simulink model "Pacemaker_Assignment_2_Final"  (R2018b)
settings: Solver=FixedStepAuto  StartTime=0.0  StopTime=inf  FixedStep=1e-3  RelTol=1e-3  EnableMultiTasking=on
undefined symbols (not defined in the file): D0, D1, D10, D11, D12, D13, D2, D3, D4, D5, D6, D7, D8, D9, PTA0, PTA1, PTA2, PTB23, PTB9, PTC16, PTC17, PTC2, PTC3, PTC4, PTD0, PTD1, PTD2, PTD3
libraries: frdmk64flib x20, dspstat3 x1
(part 2 of 2)

== stateflow chart Pacemaker_Assignment_2_Final/Pacing ==
  state VOO
    note: VOO just paces the ventricle at a rate predetermined by the LRL. Charging and discharging are seperate states simply for the sake of making the model visually similar
        | to the pacemaker shield explained doc's description of pulsing
    state Start
      entry:
      VOO_Charge_Time = 60000/Lower_Rate_Limit - Ventricular_Pulse_Width;
    state Pacing_Ventricle
      entry:
      PACE_CHARGE_CTRL = false;
      PACE_GND_CTRL = true;
      ATR_PACE_CTRL = false;
      ATR_GND_CTRL = false;
      Z_ATR_CTRL = false;
      Z_VENT_CTRL = false;
      VENT_GND_CTRL = false;
      VENT_PACE_CTRL = true;
    state Discharge_Ventricle
      entry:
      PACE_GND_CTRL = true;
      VENT_PACE_CTRL = false;
      Z_ATR_CTRL = false;
      Z_VENT_CTRL = false;
      ATR_PACE_CTRL = false;
      ATR_GND_CTRL = false;
      VENT_GND_CTRL = true;
    state Charging_Ventricle
      entry:
      ATR_PACE_CTRL = false;
      VENT_PACE_CTRL = false;
      PACING_REF_PWM = Ventricular_PWM;
      PACE_CHARGE_CTRL = true;
    (default) -> VOO.Start
    VOO.Start -> VOO.Charging_Ventricle
    VOO.Charging_Ventricle -> VOO.Pacing_Ventricle : [after(VOO_Charge_Time, msec)]
    VOO.Pacing_Ventricle -> VOO.Discharge_Ventricle : [after(Ventricular_Pulse_Width, msec)]
    VOO.Discharge_Ventricle -> VOO.Charging_Ventricle
  state AAI
    note: AAI still paces the atrium like AOO did, but must also inhibit the pacemaker if it senses a natural pace after the atrial refractory period has been reached since the last pulse (paced/natural)
    state Start
      entry:
      AAI_Charge_Time = 60000/Lower_Rate_Limit - Atrial_Pulse_Width;
      FRONTEND_CTRL = true;
    state Pacing_Atrial
      entry:
      PACE_CHARGE_CTRL = false;
      PACE_GND_CTRL = true;
      ATR_PACE_CTRL = true;
      ATR_GND_CTRL = false;
      Z_ATR_CTRL = false;
      Z_VENT_CTRL = false;
      VENT_GND_CTRL = false;
      VENT_PACE_CTRL = false;
    state Discharge_Atrial
      entry:
      PACE_GND_CTRL = true;
      VENT_PACE_CTRL = false;
      Z_ATR_CTRL = false;
      Z_VENT_CTRL = false;
      ATR_PACE_CTRL = false;
      ATR_GND_CTRL = true;
      VENT_GND_CTRL = false;
    state Charging_Atrial
      entry:
      ATR_PACE_CTRL = false;
      VENT_PACE_CTRL = false;
      PACING_REF_PWM = Atrial_PWM;
      PACE_CHARGE_CTRL = true;
    (default) -> AAI.Start
    AAI.Charging_Atrial -> AAI.Discharge_Atrial [order 2] : [Atrial_Pulse && after(ARP, msec)]
    AAI.Start -> AAI.Charging_Atrial
    AAI.Charging_Atrial -> AAI.Pacing_Atrial [order 1] : [after(AAI_Charge_Time, msec)]
    AAI.Pacing_Atrial -> AAI.Discharge_Atrial : [after(Atrial_Pulse_Width, msec)]
    AAI.Discharge_Atrial -> AAI.Charging_Atrial
  state VVI
    note: VVI still paces the atrium like VOO did, but must also inhibit the pacemaker if it senses a natural pace after the ventricular refractory period has been reached since the last pulse (paced/natural)
    state Start
      entry:
      VVI_Charge_Time = 60000/Lower_Rate_Limit - Ventricular_Pulse_Width;
      FRONTEND_CTRL = true;
    state Pacing_Ventricle
      entry:
      PACE_CHARGE_CTRL = false;
      PACE_GND_CTRL = true;
      ATR_PACE_CTRL = false;
      ATR_GND_CTRL = false;
      Z_ATR_CTRL = false;
      Z_VENT_CTRL = false;
      VENT_GND_CTRL = false;
      VENT_PACE_CTRL = true;
    state Discharge_Ventricle
      entry:
      PACE_GND_CTRL = true;
      VENT_PACE_CTRL = false;
      Z_ATR_CTRL = false;
      Z_VENT_CTRL = false;
      ATR_PACE_CTRL = false;
      ATR_GND_CTRL = false;
      VENT_GND_CTRL = true;
    state Charging_Ventricle
      entry:
      ATR_PACE_CTRL = false;
      VENT_PACE_CTRL = false;
      PACING_REF_PWM = Ventricular_PWM;
      PACE_CHARGE_CTRL = true;
    (default) -> VVI.Start
    VVI.Charging_Ventricle -> VVI.Discharge_Ventricle [order 2] : [Ventricular_Pulse && after(VRP, msec)]
    VVI.Start -> VVI.Charging_Ventricle
    VVI.Pacing_Ventricle -> VVI.Discharge_Ventricle : [after(Ventricular_Pulse_Width, msec)]
    VVI.Charging_Ventricle -> VVI.Pacing_Ventricle [order 1] : [after(VVI_Charge_Time, msec)]
    VVI.Discharge_Ventricle -> VVI.Charging_Ventricle
  note: Mode
      | Enum
      |
      | AOO
      | 1
      |
      | VOO
      | 2
      |
      | AAI
      | 3
      |
      | VVI
      | 4
      |
      | DOO
      | 5
      |
      | AOOR
      | 6
      |
      | VOOR
      | 7
      |
      | AAIR
      | 8
      |
      | VVIR
      | 9
      |
      | DOOR
      | 10
  state AOO
    note: AOO just paces the atrium at a rate predetermined by the LRL. Charging and discharging are seperate states simply for the sake of making the model visually similar
        | to the pacemaker shield explained doc's description of pulsing
    state Start
      entry:
      AOO_Charge_Time = 60000/Lower_Rate_Limit - Atrial_Pulse_Width;
    state Pacing_Atrium
      entry:
      PACE_CHARGE_CTRL = false;
      PACE_GND_CTRL = true;
      ATR_PACE_CTRL = true;
      ATR_GND_CTRL = false;
      Z_ATR_CTRL = false;
      Z_VENT_CTRL = false;
      VENT_GND_CTRL = false;
      VENT_PACE_CTRL = false;
    state Discharge_Atrium
      entry:
      PACE_GND_CTRL = true;
      VENT_PACE_CTRL = false;
      Z_ATR_CTRL = false;
      Z_VENT_CTRL = false;
      ATR_PACE_CTRL = false;
      ATR_GND_CTRL = true;
      VENT_GND_CTRL = false;
    state Charging_Atrium
      entry:
      ATR_PACE_CTRL = false;
      VENT_PACE_CTRL = false;
      PACING_REF_PWM = Atrial_PWM;
      PACE_CHARGE_CTRL = true;
    (default) -> AOO.Start
    AOO.Start -> Charging_Atrium
    Charging_Atrium -> Pacing_Atrium : [after(AOO_Charge_Time, msec)]
    Pacing_Atrium -> Discharge_Atrium : [after(Atrial_Pulse_Width, msec)]
    Discharge_Atrium -> Charging_Atrium
  state DOO
    state Start
      entry:
      DOO_Charge_Time = 60000/Lower_Rate_Limit - Fixed_AV_Delay - Ventricular_Pulse_Width;
      DOO_AV_Delay = Fixed_AV_Delay - Atrial_Pulse_Width;
      %Fixed AV Delay is from start of atrial pulse to start of ventricular pulse (must include atrial pulse width time)
    note: DOO pulses the atrium and ventricle using the LRL and Fixed AV delay for timing. The mode
        | simply transitions from pacing the ventricle to pacing the atrium and then repeats. For this mode
        | pulse amplitude sent can vary for the chambers so it must be changed based on the chamber.
    state Pacing_Ventricle
      entry:
      PACE_CHARGE_CTRL = false;
      PACE_GND_CTRL = true;
      ATR_PACE_CTRL = false;
      ATR_GND_CTRL = false;
      Z_ATR_CTRL = false;
      Z_VENT_CTRL = false;
      VENT_GND_CTRL = false;
      VENT_PACE_CTRL = true;
    state Discharge_Ventricle
      entry:
      PACE_GND_CTRL = true;
      VENT_PACE_CTRL = false;
      Z_ATR_CTRL = false;
      Z_VENT_CTRL = false;
      ATR_PACE_CTRL = false;
      ATR_GND_CTRL = false;
      VENT_GND_CTRL = true;
    state Charging_Ventricle
      entry:
      ATR_PACE_CTRL = false;
      VENT_PACE_CTRL = false;
      PACING_REF_PWM = Ventricular_PWM;
      PACE_CHARGE_CTRL = true;
    state Discharge_Atrial
      entry:
      PACE_GND_CTRL = true;
      VENT_PACE_CTRL = false;
      Z_ATR_CTRL = false;
      Z_VENT_CTRL = false;
      ATR_PACE_CTRL = false;
      ATR_GND_CTRL = true;
      VENT_GND_CTRL = false;
    state Pacing_Atrial
      entry:
      PACE_CHARGE_CTRL = false;
      PACE_GND_CTRL = true;
      ATR_PACE_CTRL = true;
      ATR_GND_CTRL = false;
      Z_ATR_CTRL = false;
      Z_VENT_CTRL = false;
      VENT_GND_CTRL = false;
      VENT_PACE_CTRL = false;
    state Charging_Atrial
      entry:
      ATR_PACE_CTRL = false;
      VENT_PACE_CTRL = false;
      PACING_REF_PWM = Atrial_PWM;
      PACE_CHARGE_CTRL = true;
    (default) -> DOO.Start
    DOO.Start -> DOO.Charging_Ventricle
    DOO.Charging_Ventricle -> DOO.Pacing_Ventricle : [after(DOO_AV_Delay, msec)]
    DOO.Pacing_Ventricle -> DOO.Discharge_Ventricle : [after(Ventricular_Pulse_Width, msec)]
    DOO.Discharge_Atrial -> DOO.Charging_Ventricle
    DOO.Discharge_Ventricle -> DOO.Charging_Atrial
    DOO.Pacing_Atrial -> DOO.Discharge_Atrial : [after(Atrial_Pulse_Width, msec)]
    DOO.Charging_Atrial -> DOO.Pacing_Atrial : [after(DOO_Charge_Time, msec)]
  state Mode %Go to mode (allows mode transition by serial)
    entry: %Set PWM values, range in rates
    Atrial_PWM = 100*Atrial_Amplitude/5;
    Ventricular_PWM = 100*Ventricular_Amplitude/5;
    Rate_Range = Max_Sensor_Rate - Lower_Rate_Limit;
    K = 3; %Arbitrary Constant (Range of Activity at RF = 1)
    ATR_PACE_CTRL = false;
    VENT_PACE_CTRL = false;
  state DOOR
    note: Rate Increase = (MSR-LRL)/Reaction Time
        | Rate Decrease = (MSR-LRL)/Recovery Time
        | Rate Range = MSR - LRL
        | Target Rate = LRL + Response Factor * (MSR - LRL)/K*(Activity - Activity Threshold)
        | Target Constant = Response Factor * Rate Range / K
        | Target Rate = LRL + Target Constant * (Activity - Activity Threshold)
    state Pacing_Ventricle
      entry:
      PACE_CHARGE_CTRL = false;
      PACE_GND_CTRL = true;
      ATR_PACE_CTRL = false;
      ATR_GND_CTRL = false;
      Z_ATR_CTRL = false;
      Z_VENT_CTRL = false;
      VENT_GND_CTRL = false;
      VENT_PACE_CTRL = true;
    state Discharge_Ventricle
      entry:
      PACE_GND_CTRL = true;
      VENT_PACE_CTRL = false;
      Z_ATR_CTRL = false;
      Z_VENT_CTRL = false;
      ATR_PACE_CTRL = false;
      ATR_GND_CTRL = false;
      VENT_GND_CTRL = true;
    state Charging_Atrial
      entry:
      ATR_PACE_CTRL = false;
      VENT_PACE_CTRL = false;
      PACING_REF_PWM = Atrial_PWM;
      PACE_CHARGE_CTRL = true;
    state Start
      entry:
      DOOR_AV_Delay = Fixed_AV_Delay - Atrial_Pulse_Width;
      %Fixed AV Delay is from start of atrial pulse to start of ventricular pulse (must include atrial pulse width time)
      DOOR_Rate = Lower_Rate_Limit;
      DOOR_Target = Lower_Rate_Limit; %Need to initialize
      Rate_Increase = (Rate_Range) / Reaction_Time;
      Rate_Decrease = (Rate_Range) / Recovery_Time;
      Target_Constant = Response_Factor * Rate_Range/K;
    state Charging_Ventricle
      entry:
      ATR_PACE_CTRL = false;
      VENT_PACE_CTRL = false;
      PACING_REF_PWM = Ventricular_PWM;
      PACE_CHARGE_CTRL = true;
      DOOR_Interval = 60000/DOOR_Rate - DOOR_AV_Delay - Ventricular_Pulse_Width;
      %Interval is calculated every loop incase rate changes
    state Pacing_Atrial
      entry:
      PACE_CHARGE_CTRL = false;
      PACE_GND_CTRL = true;
      ATR_PACE_CTRL = true;
      ATR_GND_CTRL = false;
      Z_ATR_CTRL = false;
      Z_VENT_CTRL = false;
      VENT_GND_CTRL = false;
      VENT_PACE_CTRL = false;
    state Discharge_Atrial
      entry:
      PACE_GND_CTRL = true;
      VENT_PACE_CTRL = false;
      Z_ATR_CTRL = false;
      Z_VENT_CTRL = false;
      ATR_PACE_CTRL = false;
      ATR_GND_CTRL = true;
      VENT_GND_CTRL = false;
    state Active
      entry:
      DOOR_Target = Lower_Rate_Limit + Target_Constant*(Activity - Activity_Threshold);
      DOOR_Target = min(Max_Sensor_Rate, DOOR_Target);
      %Ensure target rate is below max sensor rate
      Smooth_Rate_Increase = DOOR_Rate * Rate_Smoothing_Up/100;
    state Increase_Rate
      entry:
      DOOR_Increase = min(Smooth_Rate_Increase, Rate_Increase);
      %Applies Rate Smoothing
      DOOR_Increase = DOOR_Increase * 60/DOOR_Rate;
      DOOR_Rate = DOOR_Rate + DOOR_Increase;
    state Rate_Adaptive
      %Determines branch based on activity relative to threshold
      %Must be 0.1g above or below threshold to adjust rate
    state Limit_Rate
      %Ensure rate is between target and LRL
      entry:
      DOOR_Rate = min(DOOR_Target, DOOR_Rate);
      DOOR_Rate = max(Lower_Rate_Limit, DOOR_Rate);
    state Inactive
      entry:
      Smooth_Rate_Decrease = AAIR_Rate * Rate_Smoothing_Down/100;
    state Decrease_Rate
      entry:
      DOOR_Decrease = min(Smooth_Rate_Decrease, Rate_Decrease);
      %Applies Rate Smoothing
      DOOR_Decrease = DOOR_Decrease * 60/DOOR_Rate;
      DOOR_Rate = DOOR_Rate - DOOR_Decrease;
    (default) -> DOOR.Start
    DOOR.Charging_Ventricle -> DOOR.Pacing_Ventricle : [after(DOOR_AV_Delay, msec)]
    DOOR.Discharge_Ventricle -> DOOR.Charging_Atrial
    DOOR.Pacing_Ventricle -> DOOR.Discharge_Ventricle : [after(Ventricular_Pulse_Width, msec)]
    DOOR.Charging_Atrial -> DOOR.Pacing_Atrial : [after(DOOR_Interval, msec)]
    DOOR.Start -> DOOR.Charging_Ventricle
    DOOR.Limit_Rate -> DOOR.Charging_Ventricle
    DOOR.Pacing_Atrial -> DOOR.Discharge_Atrial : [after(Atrial_Pulse_Width, msec)]
    DOOR.Discharge_Atrial -> DOOR.Rate_Adaptive
    DOOR.Active -> DOOR.Increase_Rate
    DOOR.Rate_Adaptive -> DOOR.Active [order 1] : [Activity > (Activity_Threshold + 0.1)]
    DOOR.Increase_Rate -> DOOR.Limit_Rate
    DOOR.Rate_Adaptive -> DOOR.Limit_Rate [order 3] : [(Activity <= (Activity_Threshold + 0.1)) && (Activity >= (Activity_Threshold - 0.1))]
    DOOR.Rate_Adaptive -> DOOR.Inactive [order 2] : [Activity < (Activity_Threshold - 0.1)]
    DOOR.Decrease_Rate -> DOOR.Limit_Rate
    DOOR.Inactive -> DOOR.Decrease_Rate
  state AOOR
    note: Rate Increase = (MSR-LRL)/Reaction Time
        | Rate Decrease = (MSR-LRL)/Recovery Time
        | Rate Range = MSR - LRL
        | Target Rate = LRL + Response Factor * (MSR - LRL)/K*(Activity - Activity Threshold)
        | Target Constant = Response Factor * Rate Range / K
        | Target Rate = LRL + Target Constant * (Activity - Activity Threshold)
    state Start
      entry:
      AOOR_Rate = Lower_Rate_Limit;
      AOOR_Target = Lower_Rate_Limit; %Need to initialize
      Rate_Increase = (Rate_Range) / Reaction_Time;
      Rate_Decrease = (Rate_Range) / Recovery_Time;
      Target_Constant = Response_Factor * Rate_Range/K;
    state Pacing_Atrial
      entry:
      PACE_CHARGE_CTRL = false;
      PACE_GND_CTRL = true;
      ATR_PACE_CTRL = true;
      ATR_GND_CTRL = false;
      Z_ATR_CTRL = false;
      Z_VENT_CTRL = false;
      VENT_GND_CTRL = false;
      VENT_PACE_CTRL = false;
    state Discharge_Atrial
      entry:
      PACE_GND_CTRL = true;
      VENT_PACE_CTRL = false;
      Z_ATR_CTRL = false;
      Z_VENT_CTRL = false;
      ATR_PACE_CTRL = false;
      ATR_GND_CTRL = true;
      VENT_GND_CTRL = false;
    state Charging_Atrial
      entry:
      ATR_PACE_CTRL = false;
      VENT_PACE_CTRL = false;
      PACING_REF_PWM = Atrial_PWM;
      PACE_CHARGE_CTRL = true;
      AOOR_Interval = 60000/AOOR_Rate - Atrial_Pulse_Width;
      %Interval is calculated every loop incase rate changes
    state Active
      entry:
      AOOR_Target = Lower_Rate_Limit + Target_Constant*(Activity - Activity_Threshold);
      AOOR_Target = min(Max_Sensor_Rate, AOOR_Target);
      %Ensure target rate is below max sensor rate
      Smooth_Rate_Increase = AOOR_Rate * Rate_Smoothing_Up/100;
    state Increase_Rate
      entry:
      AOOR_Increase = min(Smooth_Rate_Increase, Rate_Increase);
      %Applies Rate Smoothing
      AOOR_Increase = AOOR_Increase * 60/AOOR_Rate;
      AOOR_Rate = AOOR_Rate + AOOR_Increase;
    state Rate_Adaptive
      %Determines branch based on activity relative to threshold
      %Must be 0.1g above or below threshold to adjust rate
    state Limit_Rate
      %Ensure rate is between target and LRL
      entry:
      AOOR_Rate = min(AOOR_Target, AOOR_Rate);
      AOOR_Rate = max(Lower_Rate_Limit, AOOR_Rate);
    state Inactive
      entry:
      Smooth_Rate_Decrease = AAIR_Rate * Rate_Smoothing_Down/100;
    state Decrease_Rate
      entry:
      AOOR_Decrease = min(Smooth_Rate_Decrease, Rate_Decrease);
      %Applies Rate Smoothing
      AOOR_Decrease = AOOR_Decrease * 60/AOOR_Rate;
      AOOR_Rate = AOOR_Rate - AOOR_Decrease;
    (default) -> AOOR.Start
    AOOR.Start -> AOOR.Charging_Atrial
    AOOR.Charging_Atrial -> AOOR.Pacing_Atrial : [after(AOOR_Interval, msec)]
    AOOR.Pacing_Atrial -> AOOR.Discharge_Atrial : [after(Atrial_Pulse_Width, msec)]
    AOOR.Limit_Rate -> AOOR.Charging_Atrial
    AOOR.Discharge_Atrial -> AOOR.Rate_Adaptive
    AOOR.Active -> AOOR.Increase_Rate
    AOOR.Rate_Adaptive -> AOOR.Active [order 1] : [Activity > (Activity_Threshold + 0.1)]
    AOOR.Increase_Rate -> AOOR.Limit_Rate
    AOOR.Rate_Adaptive -> AOOR.Limit_Rate [order 3] : [(Activity <= (Activity_Threshold + 0.1)) && (Activity >= (Activity_Threshold - 0.1))]
    AOOR.Rate_Adaptive -> AOOR.Inactive [order 2] : [Activity < (Activity_Threshold - 0.1)]
    AOOR.Decrease_Rate -> AOOR.Limit_Rate
    AOOR.Inactive -> AOOR.Decrease_Rate
  note: This is where common variables between modes are set, and the pacemaker mode is determined. This design allows hiding of the mode implementations and allows a more modular device. This setup also ensures that a mode is left once the mode changes (==mode to enter, ~= mode to exit).
  state VVIR
    state Start
      entry:
      VVIR_Rate = Lower_Rate_Limit;
      VVIR_Target = Lower_Rate_Limit; %Need to initialize
      Rate_Increase = (Rate_Range) / Reaction_Time;
      Rate_Decrease = (Rate_Range) / Recovery_Time;
      Target_Constant = Response_Factor * Rate_Range/K;
      FRONTEND_CTRL = true;
    note: Rate Increase = (MSR-LRL)/Reaction Time
        | Rate Decrease = (MSR-LRL)/Recovery Time
        | Rate Range = MSR - LRL
        | Target Rate = LRL + Response Factor * (MSR - LRL)/K*(Activity - Activity Threshold)
        | Target Constant = Response Factor * Rate Range / K
        | Target Rate = LRL + Target Constant * (Activity - Activity Threshold)
    state Charging_Ventricle
      entry:
      ATR_PACE_CTRL = false;
      VENT_PACE_CTRL = false;
      PACING_REF_PWM = Ventricular_PWM;
      PACE_CHARGE_CTRL = true;
      VVIR_Interval = 60000/VVIR_Rate - Ventricular_Pulse_Width;
      %Interval is calculated every loop incase rate changes
      sensed = false;
    state Pacing_Ventricle
      entry:
      PACE_CHARGE_CTRL = false;
      PACE_GND_CTRL = true;
      ATR_PACE_CTRL = false;
      ATR_GND_CTRL = false;
      Z_ATR_CTRL = false;
      Z_VENT_CTRL = false;
      VENT_GND_CTRL = false;
      VENT_PACE_CTRL = true;
    state Discharge_Ventricle
      entry:
      PACE_GND_CTRL = true;
      VENT_PACE_CTRL = false;
      Z_ATR_CTRL = false;
      Z_VENT_CTRL = false;
      ATR_PACE_CTRL = false;
      ATR_GND_CTRL = false;
      VENT_GND_CTRL = true;
    state Increase_Rate_Sensed
      entry:
      VVIR_Increase = min(Smooth_Rate_Increase, Rate_Increase);
      %Applies Rate Smoothing
      VVIR_Increase = VVIR_Increase * VRP/1000;
      VVIR_Rate = VVIR_Rate + VVIR_Increase;
    state Active
      entry:
      VVIR_Target = Lower_Rate_Limit + Target_Constant*(Activity - Activity_Threshold);
      VVIR_Target = min(Max_Sensor_Rate, VVIR_Target);
      %Ensure target rate is below max sensor rate
      Smooth_Rate_Increase = VVIR_Rate * Rate_Smoothing_Up/100;
    state Increase_Rate_Paced
      entry:
      VVIR_Increase = min(Smooth_Rate_Increase, Rate_Increase);
      %Applies Rate Smoothing
      VVIR_Increase = VVIR_Increase * 60/VVIR_Rate;
      VVIR_Rate = VVIR_Rate + VVIR_Increase;
    state Rate_Adaptive
      %Determines branch based on activity relative to threshold
      %Must be 0.1g above or below threshold to adjust rate
    state Limit_Rate
      %Ensure rate is between target and LRL
      entry:
      VVIR_Rate = min(VVIR_Target, VVIR_Rate);
      VVIR_Rate = max(Lower_Rate_Limit, VVIR_Rate);
    state Decrease_Rate_Sensed
      entry:
      VVIR_Decrease = min(Smooth_Rate_Decrease, Rate_Decrease);
      %Applies Rate Smoothing
      VVIR_Decrease = VVIR_Decrease * VRP/1000;
      VVIR_Rate = VVIR_Rate - VVIR_Decrease;
    state Inactive
      entry:
      Smooth_Rate_Decrease = VVIR_Rate * Rate_Smoothing_Down/100;
    state Decrease_Rate_Paced
      entry:
      VVIR_Decrease = min(Smooth_Rate_Decrease, Rate_Decrease);
      %Applies Rate Smoothing
      VVIR_Decrease = VVIR_Decrease * 60/VVIR_Rate;
      VVIR_Rate = VVIR_Rate - VVIR_Decrease;
    (default) -> VVIR.Start
    VVIR.Start -> VVIR.Charging_Ventricle
    VVIR.Charging_Ventricle -> VVIR.Discharge_Ventricle [order 1] : [Ventricular_Pulse && after(VRP, msec)]{sensed = true;}
    VVIR.Charging_Ventricle -> VVIR.Pacing_Ventricle [order 2] : [after(VVIR_Interval, msec)]
    VVIR.Pacing_Ventricle -> VVIR.Discharge_Ventricle : [after(Ventricular_Pulse_Width, msec)]
    VVIR.Limit_Rate -> VVIR.Charging_Ventricle
    VVIR.Discharge_Ventricle -> VVIR.Rate_Adaptive
    VVIR.Active -> VVIR.Increase_Rate_Sensed [order 1] : [sensed]
    VVIR.Increase_Rate_Sensed -> VVIR.Limit_Rate
    VVIR.Rate_Adaptive -> VVIR.Active [order 1] : [Activity > (Activity_Threshold + 0.1)]
    VVIR.Active -> VVIR.Increase_Rate_Paced [order 2] : [~sensed]
    VVIR.Increase_Rate_Paced -> VVIR.Limit_Rate
    VVIR.Rate_Adaptive -> VVIR.Limit_Rate [order 3] : [(Activity <= (Activity_Threshold + 0.1)) && (Activity >= (Activity_Threshold - 0.1))]
    VVIR.Decrease_Rate_Sensed -> VVIR.Limit_Rate
    VVIR.Rate_Adaptive -> VVIR.Inactive [order 2] : [Activity < (Activity_Threshold - 0.1)]
    VVIR.Decrease_Rate_Paced -> VVIR.Limit_Rate
    VVIR.Inactive -> VVIR.Decrease_Rate_Sensed [order 2] : [sensed]
    VVIR.Inactive -> VVIR.Decrease_Rate_Paced [order 1] : [~sensed]
  state AAIR
    note: Rate Increase = (MSR-LRL)/Reaction Time
        | Rate Decrease = (MSR-LRL)/Recovery Time
        | Rate Range = MSR - LRL
        | Target Rate = LRL + Response Factor * (MSR - LRL)/K*(Activity - Activity Threshold)
        | Target Constant = Response Factor * Rate Range / K
        | Target Rate = LRL + Target Constant * (Activity - Activity Threshold)
    state Start
      entry:
      AAIR_Rate = Lower_Rate_Limit;
      AAIR_Target = Lower_Rate_Limit; %Need to initialize
      Rate_Increase = (Rate_Range) / Reaction_Time;
      Rate_Decrease = (Rate_Range) / Recovery_Time;
      Target_Constant = Response_Factor * Rate_Range/K;
      FRONTEND_CTRL = true;
    state Charging_Atrial
      entry:
      ATR_PACE_CTRL = false;
      VENT_PACE_CTRL = false;
      PACING_REF_PWM = Atrial_PWM;
      PACE_CHARGE_CTRL = true;
      AAIR_Interval = 60000/AAIR_Rate - Atrial_Pulse_Width;
      %Interval is calculated every loop incase rate changes
      sensed = false;
    state Pacing_Atrial
      entry:
      PACE_CHARGE_CTRL = false;
      PACE_GND_CTRL = true;
      ATR_PACE_CTRL = true;
      ATR_GND_CTRL = false;
      Z_ATR_CTRL = false;
      Z_VENT_CTRL = false;
      VENT_GND_CTRL = false;
      VENT_PACE_CTRL = false;
    state Discharge_Atrial
      entry:
      PACE_GND_CTRL = true;
      VENT_PACE_CTRL = false;
      Z_ATR_CTRL = false;
      Z_VENT_CTRL = false;
      ATR_PACE_CTRL = false;
      ATR_GND_CTRL = true;
      VENT_GND_CTRL = false;
    state Increase_Rate_Sensed
      entry:
      AAIR_Increase = min(Smooth_Rate_Increase, Rate_Increase);
      %Applies Rate Smoothing
      AAIR_Increase = AAIR_Increase * ARP/1000;
      AAIR_Rate = AAIR_Rate + AAIR_Increase;
    state Active
      entry:
      AAIR_Target = Lower_Rate_Limit + Target_Constant*(Activity - Activity_Threshold);
      AAIR_Target = min(Max_Sensor_Rate, AAIR_Target);
      %Ensure target rate is below max sensor rate
      Smooth_Rate_Increase = AAIR_Rate * Rate_Smoothing_Up/100;
    state Increase_Rate_Paced
      entry:
      AAIR_Increase = min(Smooth_Rate_Increase, Rate_Increase);
      %Applies Rate Smoothing
      AAIR_Increase = AAIR_Increase * 60/AAIR_Rate;
      AAIR_Rate = AAIR_Rate + AAIR_Increase;
    state Rate_Adaptive
      %Determines branch based on activity relative to threshold
      %Must be 0.1g above or below threshold to adjust rate
    state Limit_Rate
      %Ensure rate is between target and LRL
      entry:
      AAIR_Rate = min(AAIR_Target, AAIR_Rate);
      AAIR_Rate = max(Lower_Rate_Limit, AAIR_Rate);
    state Decrease_Rate_Sensed
      entry:
      AAIR_Decrease = min(Smooth_Rate_Decrease, Rate_Decrease);
      %Applies Rate Smoothing
      AAIR_Decrease = AAIR_Decrease * ARP/1000;
      AAIR_Rate = AAIR_Rate - AAIR_Decrease;
    state Inactive
      entry:
      Smooth_Rate_Decrease = AAIR_Rate * Rate_Smoothing_Down/100;
    state Decrease_Rate_Paced
      entry:
      AAIR_Decrease = min(Smooth_Rate_Decrease, Rate_Decrease);
      %Applies Rate Smoothing
      AAIR_Decrease = AAIR_Decrease * 60/AAIR_Rate;
      AAIR_Rate = AAIR_Rate - AAIR_Decrease;
    (default) -> AAIR.Start
    AAIR.Charging_Atrial -> AAIR.Discharge_Atrial [order 1] : [Atrial_Pulse && after(ARP, msec)]{sensed = true;}
    AAIR.Start -> AAIR.Charging_Atrial
    AAIR.Charging_Atrial -> AAIR.Pacing_Atrial [order 2] : [after(AAIR_Interval, msec)]
    AAIR.Pacing_Atrial -> AAIR.Discharge_Atrial : [after(Atrial_Pulse_Width, msec)]
    AAIR.Limit_Rate -> AAIR.Charging_Atrial
    AAIR.Discharge_Atrial -> AAIR.Rate_Adaptive
    AAIR.Active -> AAIR.Increase_Rate_Sensed [order 1] : [sensed]
    AAIR.Increase_Rate_Sensed -> AAIR.Limit_Rate
    AAIR.Rate_Adaptive -> AAIR.Active [order 1] : [Activity > (Activity_Threshold + 0.1)]
    AAIR.Active -> AAIR.Increase_Rate_Paced [order 2] : [~sensed]
    AAIR.Increase_Rate_Paced -> AAIR.Limit_Rate
    AAIR.Rate_Adaptive -> AAIR.Limit_Rate [order 3] : [(Activity <= (Activity_Threshold + 0.1)) && (Activity >= (Activity_Threshold - 0.1))]
    AAIR.Decrease_Rate_Sensed -> AAIR.Limit_Rate
    AAIR.Rate_Adaptive -> AAIR.Inactive [order 2] : [Activity < (Activity_Threshold - 0.1)]
    AAIR.Decrease_Rate_Paced -> AAIR.Limit_Rate
    AAIR.Inactive -> AAIR.Decrease_Rate_Sensed [order 2] : [sensed]
    AAIR.Inactive -> AAIR.Decrease_Rate_Paced [order 1] : [~sensed]
  state VOOR
    state Start
      entry:
      VOOR_Rate = Lower_Rate_Limit;
      VOOR_Target = Lower_Rate_Limit; %Need to initialize
      Rate_Increase = (Rate_Range) / Reaction_Time;
      Rate_Decrease = (Rate_Range) / Recovery_Time;
      Target_Constant = Response_Factor * Rate_Range/K;
    note: Rate Increase = (MSR-LRL)/Reaction Time
        | Rate Decrease = (MSR-LRL)/Recovery Time
        | Rate Range = MSR - LRL
        | Target Rate = LRL + Response Factor * (MSR - LRL)/K*(Activity - Activity Threshold)
        | Target Constant = Response Factor * Rate Range / K
        | Target Rate = LRL + Target Constant * (Activity - Activity Threshold)
    state Pacing_Ventricle
      entry:
      PACE_CHARGE_CTRL = false;
      PACE_GND_CTRL = true;
      ATR_PACE_CTRL = false;
      ATR_GND_CTRL = false;
      Z_ATR_CTRL = false;
      Z_VENT_CTRL = false;
      VENT_GND_CTRL = false;
      VENT_PACE_CTRL = true;
    state Discharge_Ventricle
      entry:
      PACE_GND_CTRL = true;
      VENT_PACE_CTRL = false;
      Z_ATR_CTRL = false;
      Z_VENT_CTRL = false;
      ATR_PACE_CTRL = false;
      ATR_GND_CTRL = false;
      VENT_GND_CTRL = true;
    state Charging_Ventricle
      entry:
      ATR_PACE_CTRL = false;
      VENT_PACE_CTRL = false;
      PACING_REF_PWM = Ventricular_PWM;
      PACE_CHARGE_CTRL = true;
      VOOR_Interval = 60000/VOOR_Rate - Ventricular_Pulse_Width;
      %Interval is calculated every loop incase rate changes
    state Active
      entry:
      VOOR_Target = Lower_Rate_Limit + Target_Constant*(Activity - Activity_Threshold);
      VOOR_Target = min(Max_Sensor_Rate, VOOR_Target);
      %Ensure target rate is below max sensor rate
      Smooth_Rate_Increase = VOOR_Rate * Rate_Smoothing_Up/100;
    state Increase_Rate
      entry:
      VOOR_Increase = min(Smooth_Rate_Increase, Rate_Increase);
      %Applies Rate Smoothing
      VOOR_Increase = VOOR_Increase * 60/VOOR_Rate;
      VOOR_Rate = VOOR_Rate + VOOR_Increase;
    state Rate_Adaptive
      %Determines branch based on activity relative to threshold
      %Must be 0.1g above or below threshold to adjust rate
    state Limit_Rate
      %Ensure rate is between target and LRL
      entry:
      VOOR_Rate = min(VOOR_Target, VOOR_Rate);
      VOOR_Rate = max(Lower_Rate_Limit, VOOR_Rate);
    state Inactive
      entry:
      Smooth_Rate_Decrease = VVIR_Rate * Rate_Smoothing_Down/100;
    state Decrease_Rate
      entry:
      VOOR_Decrease = min(Smooth_Rate_Decrease, Rate_Decrease);
      %Applies Rate Smoothing
      VOOR_Decrease = VOOR_Decrease * 60/VOOR_Rate;
      VOOR_Rate = VOOR_Rate - VOOR_Decrease;
    (default) -> VOOR.Start
    VOOR.Start -> VOOR.Charging_Ventricle
    VOOR.Charging_Ventricle -> VOOR.Pacing_Ventricle : [after(VOOR_Interval, msec)]
    VOOR.Pacing_Ventricle -> VOOR.Discharge_Ventricle : [after(Ventricular_Pulse_Width, msec)]
    VOOR.Limit_Rate -> VOOR.Charging_Ventricle
    VOOR.Discharge_Ventricle -> VOOR.Rate_Adaptive
    VOOR.Active -> VOOR.Increase_Rate
    VOOR.Rate_Adaptive -> VOOR.Active [order 1] : [Activity > (Activity_Threshold + 0.1)]
    VOOR.Increase_Rate -> VOOR.Limit_Rate
    VOOR.Rate_Adaptive -> VOOR.Limit_Rate [order 3] : [(Activity <= (Activity_Threshold + 0.1)) && (Activity >= (Activity_Threshold - 0.1))]
    VOOR.Rate_Adaptive -> VOOR.Inactive [order 2] : [Activity < (Activity_Threshold - 0.1)]
    VOOR.Decrease_Rate -> VOOR.Limit_Rate
    VOOR.Inactive -> VOOR.Decrease_Rate
  VOO -> Mode %Go to mode (allows mode transition by serial) : [Mode ~= 2]
  Mode %Go to mode (allows mode transition by serial) -> VOO [order 2] : [Mode == 2]
  AAI -> Mode %Go to mode (allows mode transition by serial) : [Mode ~= 3]
  Mode %Go to mode (allows mode transition by serial) -> AAI [order 3] : [Mode == 3]
  Mode %Go to mode (allows mode transition by serial) -> VVI [order 4] : [Mode == 4]
  VVI -> Mode %Go to mode (allows mode transition by serial) : [Mode ~= 4]
  (default) -> Mode %Go to mode (allows mode transition by serial)
  Mode %Go to mode (allows mode transition by serial) -> DOO [order 5] : [Mode == 5]
  Mode %Go to mode (allows mode transition by serial) -> AOO [order 1] : [Mode == 1]
  DOO -> Mode %Go to mode (allows mode transition by serial) : [Mode ~= 5]
  AOO -> Mode %Go to mode (allows mode transition by serial) : [Mode ~= 1]
  DOOR -> Mode %Go to mode (allows mode transition by serial) : [Mode ~= 10]
  Mode %Go to mode (allows mode transition by serial) -> AOOR [order 6] : [Mode == 6]
  Mode %Go to mode (allows mode transition by serial) -> DOOR [order 10] : [Mode == 10]
  AOOR -> Mode %Go to mode (allows mode transition by serial) : [Mode ~= 6]
  VVIR -> Mode %Go to mode (allows mode transition by serial) : [Mode ~= 9]
  Mode %Go to mode (allows mode transition by serial) -> VVIR [order 9] : [Mode == 9]
  Mode %Go to mode (allows mode transition by serial) -> AAIR [order 8] : [Mode == 8]
  AAIR -> Mode %Go to mode (allows mode transition by serial) : [Mode ~= 8]
  Mode %Go to mode (allows mode transition by serial) -> VOOR [order 7] : [Mode == 7]
  VOOR -> Mode %Go to mode (allows mode transition by serial) : [Mode ~= 7]
  data: Mode input; Lower_Rate_Limit input; Upper_Rate_Limit input; Max_Sensor_Rate input; Fixed_AV_Delay input; FRONTEND_CTRL output; PACING_REF_PWM output; ATR_PACE_CTRL output; VENT_PACE_CTRL output; PACE_CHARGE_CTRL output; PACE_GND_CTRL output; ATR_GND_CTRL output; VENT_GND_CTRL output; Z_ATR_CTRL output; Z_VENT_CTRL output; Atrial_Amplitude input; Ventricular_Amplitude input; Atrial_Pulse_Width input; Ventricular_Pulse_Width input; VRP input; ARP input; Rate_Smoothing_Up input; Rate_Smoothing_Down input; Activity_Threshold input; Reaction_Time input; Response_Factor input; Recovery_Time input; Atrial_Pulse input; Ventricular_Pulse input; Activity input; DOOR_AV_Delay local; VVI_Charge_Time local; DOO_Charge_Time local; DOO_AV_Delay local; AOO_Charge_Time local; VOO_Charge_Time local; AAI_Charge_Time local; AAIR_Increase local; DOOR_Rate local; VOOR_Rate local; VOOR_Interval local; AAIR_Decrease local; Rate_Increase local; sensed local; AOOR_Increase local; AOOR_Decrease local; AOOR_Rate local; AOOR_Interval local; VVIR_Rate local; DOOR_Interval local; Rate_Decrease local; DOOR_Increase local; DOOR_Decrease local; AAIR_Interval local; VVIR_Interval local; VVIR_Increase local; VVIR_Decrease local; AAIR_Rate local; K local; Ventricular_PWM local; Atrial_PWM local; Rate_Range local; Target_Constant local; DOOR_Target local; Smooth_Rate_Decrease local; Smooth_Rate_Increase local; AOOR_Target local; VVIR_Target local; AAIR_Target local; VOOR_Decrease local; VOOR_Increase local; VOOR_Target local

== stateflow chart Pacemaker_Assignment_2_Final/DCM Serial Inputs/Serial_Receive ==
  settings: executeAtInitialization=1
  state INITIAL
    %Values to Reset to
    entry:
    Mode = 0;
    LRL = 0;
    URL = 0;
    MSR = 0;
    FAVD = 0;
    APA = 0;
    VPA = 0;
    APW = 0;
    VPW = 0;
    ARP = 0;
    VRP = 0;
    RSU = 0;
    RSD = 0;
    AT = 0;
    ReactT = 0;
    RF = 0;
    RecovT = 0;
  state RECEIVE
    entry:
    %Serial Data is received properly
    %Values updated and scaled from DCM
    Mode = double (Serial(2));
    LRL = double (Serial(3));
    URL = double (Serial(4));
    MSR = double (Serial(5));
    FAVD = double (Serial(6))*10;
    APA = double (Serial(7))/20;
    VPA = double (Serial(8))/20;
    APW = double (Serial(9))/10;
    VPW = double (Serial(10))/10;
    ARP = double (Serial(11))*10;
    VRP = double (Serial(12))*10;
    RSU = double (Serial(13));
    RSD = double (Serial(14));
    AT = double (Serial(15));
    ReactT = double (Serial(16));
    RF = double (Serial(17));
    RecovT = double (Serial(18));
  note: Enable = 1 if the parity check fails (reset values)
  state STANDBY
    %Waiting for
    %Serial data
  note: Values are only updated when there
      | is new data and parity check passes
  note: Mode is set to 0 (off) so that if the mode is kept the same as previously, the mode will be briefly exited so that the parameters can be updated again
  (default) -> INITIAL
  RECEIVE -> STANDBY
  STANDBY -> INITIAL [order 2] : [Enable == 1]
  INITIAL -> STANDBY
  STANDBY -> RECEIVE [order 1] : [(Status == 0) && (Enable==0)]{Mode = 0}
  data: Mode output; Serial input uint8; LRL output; URL output; MSR output; FAVD output; APA output; VPA output; APW output; VPW output; ARP output; VRP output; RSU output; RSD output; AT output; ReactT output; RF output; RecovT output; Enable input; Status input
